simulink model "datatypeconversion13"  (R2015a)
settings: Solver=VariableStepDiscrete  StartTime=0.0  StopTime=10.0  RelTol=1e-3
settings Model: CovSFcnEnable=off  Creator=arnaud  LastModifiedBy=hbourbou
settings DataIOCC: SaveFormat=StructureWithTime  SignalLoggingSaveFormat=ModelDataLogs
settings OptimizationCC: ExpressionDepthLimit=2147483647
settings DebuggingCC: UnderspecifiedInitializationDetection=Classic  MergeDetectMultiDrivingBlocksExec=none  SolverPrmCheckMsg=warning  FcnCallInpInsideContextMsg=EnableAllAsWarning  StateNameClashWarn=warning
settings GRTTargetCC: CombineOutputUpdateFcns=off  GRTInterface=on

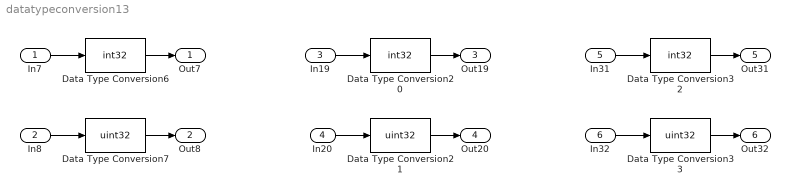
== system datatypeconversion13 ==
  In7 : Inport  OutDataTypeStr=double  PortDimensions=1
  In8 : Inport  Port=2  OutDataTypeStr=double  PortDimensions=1
  In19 : Inport  Port=3  OutDataTypeStr=single  PortDimensions=1
  In20 : Inport  Port=4  OutDataTypeStr=single  PortDimensions=1
  In31 : Inport  Port=5  OutDataTypeStr=int8  PortDimensions=1
  In32 : Inport  Port=6  OutDataTypeStr=int8  PortDimensions=1
  Data Type Conversion20 : DataTypeConversion  OutDataTypeStr=int32
  Data Type Conversion21 : DataTypeConversion  OutDataTypeStr=uint32
  Data Type Conversion32 : DataTypeConversion  OutDataTypeStr=int32
  Data Type Conversion33 : DataTypeConversion  OutDataTypeStr=uint32
  Data Type Conversion6 : DataTypeConversion  OutDataTypeStr=int32
  Data Type Conversion7 : DataTypeConversion  OutDataTypeStr=uint32
  Out7 : Outport
  Out8 : Outport  Port=2
  Out19 : Outport  Port=3
  Out20 : Outport  Port=4
  Out31 : Outport  Port=5
  Out32 : Outport  Port=6
  wires:
  In31/1 -> Data Type Conversion32/1
  In7/1 -> Data Type Conversion6/1
  Data Type Conversion33/1 -> Out32/1
  Data Type Conversion7/1 -> Out8/1
  Data Type Conversion21/1 -> Out20/1
  In32/1 -> Data Type Conversion33/1
  Data Type Conversion32/1 -> Out31/1
  Data Type Conversion6/1 -> Out7/1
  In8/1 -> Data Type Conversion7/1
  Data Type Conversion20/1 -> Out19/1
  In19/1 -> Data Type Conversion20/1
  In20/1 -> Data Type Conversion21/1
